simulink model "power_dcmotor"  (Simulink 6.0)
settings: Solver=ode23s  SolverMode=SingleTasking  StartTime=0.0  StopTime=10  RelTol=1e-3  AbsTol=1e-2
libraries: powerlib x17, powerlib_extras x1, simulink x1
settings Model: Creator=patrice  LastModifiedBy=batserve  ExtModeTrigMode=oneshot  ExtModeArmWhenConnect=off  ExtModeAutoUpdateStatusClock=off
settings DataIOCC: Decimation=5  FinalStateName=x50  InitialState=x50  LimitDataPoints=off  MaxDataPoints=500000  SaveOutput=off  TimeSaveName=t  SignalLoggingName=sigsOut
settings OptimizationCC: BlockReduction=off  BooleanDataType=off
settings DebuggingCC: CheckExecutionContextPreStartOutputMsg=on  CheckExecutionContextRuntimeOutputMsg=on  SolverPrmCheckMsg=none  IntegerOverflowMsg=none
settings HardwareCC: TargetUnknown=on
settings RTWCC: TemplateMakefile=grt_vc.tmf

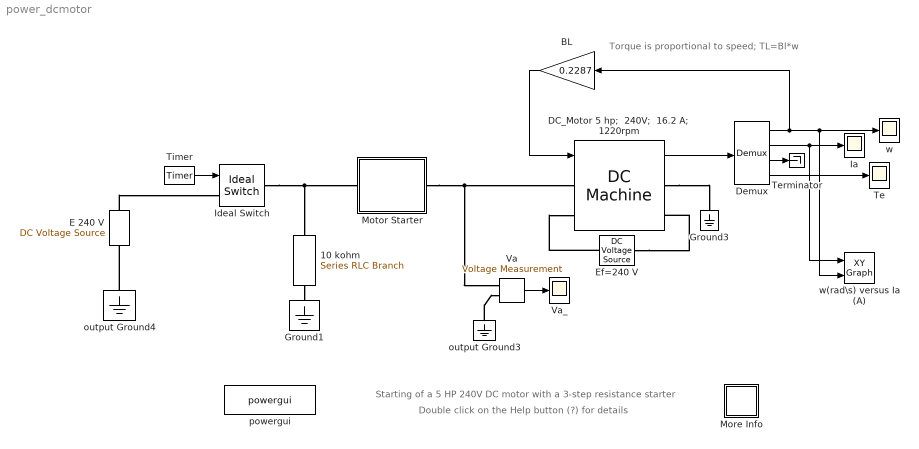
== system power_dcmotor ==
  note: Starting of a 5 HP 240V DC motor with a 3-step resistance starter
  note: Torque is proportional to speed; TL=Bl*w
  note: Double click on the Help button (?) for details
  10 kohm : powerlib/Elements/Series RLC Branch  Orientation=down  PhysicalDomain=powersysdomain  SubClassName=unknown  LeftPortType=p1  RightPortType=p1  LConnTagsString=__new0  RConnTagsString=__new0  Resistance=1e4  Inductance=0  Capacitance=inf  Measurements=None
  BL : Gain  Orientation=left  Gain=0.2287  SaturateOnIntegerOverflow=on
  DC_Motor 5 hp;  240V;  16.2 A;  1220rpm : powerlib/Machines/DC Machine  PresetModel=No  ShowDetailedParameters=on  RLa="[ 0.6  0.012]"  RLf="[ 240  120]"  Laf=1.8  J=1  Bm=0  Tf=0  w0=1
      settings: AttributesFormatString=\n
  Demux : Demux
  E 240 V : powerlib/Electrical Sources/DC Voltage Source  Description=source block  Orientation=up  Amplitude=240  Measurements=None
      settings: AttributesFormatString=\n
  Ef=240 V : powerlib/Electrical Sources/DC Voltage Source  Description=source block  Orientation=left  Amplitude=240  Measurements=None
      settings: AttributesFormatString=\n
  Ground1 : powerlib/Elements/Ground  Orientation=down  PhysicalDomain=powersysdomain  SubClassName=unknown  LeftPortType=p1  RightPortType=p1  LConnTagsString=a
  Ground3 : powerlib/Elements/Ground  Orientation=down  PhysicalDomain=powersysdomain  SubClassName=unknown  LeftPortType=p1  RightPortType=p1  LConnTagsString=a
  Ia : Scope
      settings: TickLabels=on  TimeRange=10  YMin=0  YMax=40  SaveName=Ia  DataFormat=Array  MaxDataPoints=500000
  Ideal Switch : powerlib/Power Electronics/Ideal Switch  Ron=1e-4  Lon=10e-6  IC=0  Rs=inf  Cs=0  Measurements=off
      settings: AttributesFormatString=\n
  More Info : Subsystem
      mask Display: disp('?')
  Motor Starter : Subsystem
      mask Display: disp('3 step\n\nstarter')
  Te : Scope
      settings: TickLabels=on  TimeRange=10  YMin=0  YMax=100  SaveName=Tm  DataFormat=Array  MaxDataPoints=500000
  Terminator : Terminator
  Timer : powerlib_extras/Control  Blocks/Timer  t=[0 0.5 ]  e=[0 1 ]
  Va : powerlib/Measurements/Voltage Measurement  Tag=PoWeRsYsTeMmEaSuReMeNt  PhasorSimulation=off  OutputType=Magnitude  PSBequivalent=0
  Va_ : Scope
      settings: TickLabels=on  TimeRange=10  YMin=0  YMax=300  SaveName=U_DC_mot  DataFormat=Array  MaxDataPoints=500000
  output Ground3 : powerlib/Elements/Ground  Orientation=down  PhysicalDomain=powersysdomain  SubClassName=unknown  LeftPortType=p1  RightPortType=p1  LConnTagsString=a
  output Ground4 : powerlib/Elements/Ground  Orientation=down  PhysicalDomain=powersysdomain  SubClassName=unknown  LeftPortType=p1  RightPortType=p1  LConnTagsString=a
  powergui : powerlib/powergui  Priority=2  Frange=logspace(0,3,50)  Ylog=off  Xlog=off  save=off  variable=ZData  ZoomFFT=on  StartTime=0.0  cycles=1  DisplayStyle=off  fundamental=60  FreqAxis=off  MaxFrequency=1000  frequencyindice=1  frequencyindicesteady=1  RmsSteady=1  display=off  Ts=0  methode=off  frequency=60  echomessages=off
  w : Scope
      settings: TickLabels=on  TimeRange=10  YMin=0  YMax=150  SaveName=w  DataFormat=Array  MaxDataPoints=500000
  w(rad\s) versus Ia (A) : simulink/Sinks/XY Graph  xmin=0  xmax=40  ymin=0  ymax=140  st=-1
  wires:
  Demux/4 -> Te/1
  Demux/1 -> BL/1, w/1, w(rad\s) versus Ia (A)/2
  Demux/2 -> Ia/1, w(rad\s) versus Ia (A)/1
  Demux/3 -> Terminator/1
  Timer/1 -> Ideal Switch/1
  Va/1 -> Va_/1
  DC_Motor 5 hp;  240V;  16.2 A;  1220rpm/1 -> Demux/1
  BL/1 -> DC_Motor 5 hp;  240V;  16.2 A;  1220rpm/1
  connections:
  output Ground4/LConn1 -- E 240 V/LConn1
  10 kohm/RConn1 -- Ground1/LConn1
  Ideal Switch/RConn1 -- 10 kohm/LConn1 -- Motor Starter/LConn1
  E 240 V/RConn1 -- Ideal Switch/LConn1
  Motor Starter/RConn1 -- Va/LConn1 -- DC_Motor 5 hp;  240V;  16.2 A;  1220rpm/LConn1
  DC_Motor 5 hp;  240V;  16.2 A;  1220rpm/RConn1 -- Ground3/LConn1
  output Ground3/LConn1 -- Va/LConn2
  Ef=240 V/LConn1 -- DC_Motor 5 hp;  240V;  16.2 A;  1220rpm/RConn2
  Ef=240 V/RConn1 -- DC_Motor 5 hp;  240V;  16.2 A;  1220rpm/LConn2

== system power_dcmotor/More Info ==
  note: Induced EMF:  Eo = 240-16.2*0.6 = 230.3 V
      |
      | Pe = 230.3*16.2 = 3731 W = 5.0 HP
      |
      | Field current: If = 240/240 =1 A
      |
      | Eo = w*Laf*If  --->  w = (Eo/La*If)
      | speed w = 230.3/1.8 = 127.7 rad/s = 1220 r/min
      |
      | Nominal  torque: Te = Pe/w = 3731/127.7 = 29.2 N.m
  note: DC Motor Rated Values:
  note: (Krause et al., Reference Analysis of Electric Machinery, pp. 89-92)
  note: Starting a 5 HP, 240V DC motor with a 3-step resistance starter
  note: G. Sybille (Hydro-Quebec)

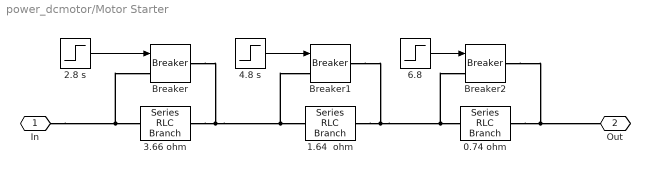
== system power_dcmotor/Motor Starter ==
  0.74 ohm : powerlib/Elements/Series RLC Branch  PhysicalDomain=powersysdomain  SubClassName=unknown  LeftPortType=p1  RightPortType=p1  LConnTagsString=__new0  RConnTagsString=__new0  Resistance=0.74  Inductance=0  Capacitance=inf  Measurements=None
  1.64  ohm : powerlib/Elements/Series RLC Branch  PhysicalDomain=powersysdomain  SubClassName=unknown  LeftPortType=p1  RightPortType=p1  LConnTagsString=__new0  RConnTagsString=__new0  Resistance=1.64  Inductance=0  Capacitance=inf  Measurements=None
  2.8 s : Step  Time=2.8  SampleTime=0  ZeroCross=off
  3.66 ohm : powerlib/Elements/Series RLC Branch  PhysicalDomain=powersysdomain  SubClassName=unknown  LeftPortType=p1  RightPortType=p1  LConnTagsString=__new0  RConnTagsString=__new0  Resistance=3.66  Inductance=0  Capacitance=inf  Measurements=None
  4.8 s : Step  Time=4.8  SampleTime=0  ZeroCross=off
  6.8 : Step  Time=6.8  SampleTime=0  ZeroCross=off
  Breaker : powerlib/Elements/Breaker  BreakerResistance=0.01  InitialState=0  SnubberResistance=inf  SnubberCapacitance=0  SwitchingTimes="[ 4/60  5/60 ]"  External=on  Measurements=None
      settings: AttributesFormatString=\n
  Breaker1 : powerlib/Elements/Breaker  BreakerResistance=0.01  InitialState=0  SnubberResistance=inf  SnubberCapacitance=0  SwitchingTimes="[ 4/60  5/60 ]"  External=on  Measurements=None
      settings: AttributesFormatString=\n
  Breaker2 : powerlib/Elements/Breaker  BreakerResistance=0.01  InitialState=0  SnubberResistance=inf  SnubberCapacitance=0  SwitchingTimes="[ 4/60  5/60 ]"  External=on  Measurements=None
      settings: AttributesFormatString=\n
  In : PMIOPort  Port=1  Side=Left
  Out : PMIOPort  Orientation=left  Port=2  Side=Right
  wires:
  4.8 s/1 -> Breaker1/1
  6.8/1 -> Breaker2/1
  2.8 s/1 -> Breaker/1
  connections:
  In/RConn1 -- 3.66 ohm/LConn1 -- Breaker/LConn1
  3.66 ohm/RConn1 -- 1.64  ohm/LConn1 -- Breaker1/LConn1 -- Breaker/RConn1
  1.64  ohm/RConn1 -- 0.74 ohm/LConn1 -- Breaker2/LConn1 -- Breaker1/RConn1
  0.74 ohm/RConn1 -- Out/RConn1 -- Breaker2/RConn1
